simulink model "corripd"  (R2025b)
settings: Solver=ode5  StartTime=0.0  StopTime=2.335  FixedStep=0.001  MaxStep=0.001  RelTol=1e-3  AbsTol=1e-3
values from neighbouring files (symbols this model uses):
  b = 5E-5    (= 5e-05)    [Constants.m]
  J = 1    [Constants.m]
  Ka = 20    [Constants.m]
  Ki = 10000    [Constants.m]
  Km = 1.36    [Constants.m]
  Kp = 50    [Constants.m]
  Kv = Kvc    [Constants.m]
settings Model: ExtModeTrigMode=oneshot  ExtModeArmWhenConnect=off  Creator=Tomás  LastModifiedBy=Tomás
settings DataIOCC: SaveFormat=Array  SignalLoggingSaveFormat=ModelDataLogs  SaveOutput=off  SaveTime=off  ReturnWorkspaceOutputs=off
settings OptimizationCC: BlockReduction=off  BooleanDataType=off
settings DebuggingCC: SaveWithParameterizedLinksMsg=none  UnderspecifiedInitializationDetection=Classic  MergeDetectMultiDrivingBlocksExec=none  SignalResolutionControl=TryResolveAllWithWarning  MultiTaskDSMMsg=warning  MultiTaskCondExecSysMsg=none  UnconnectedInputMsg=warning  UnconnectedOutputMsg=warning  UnconnectedLineMsg=warning
settings HardwareCC: TargetUnknown=on
settings ModelReferenceCC: PropagateSignalLabelsOutOfModel=off
settings GRTTargetCC: CombineOutputUpdateFcns=off  GRTInterface=on

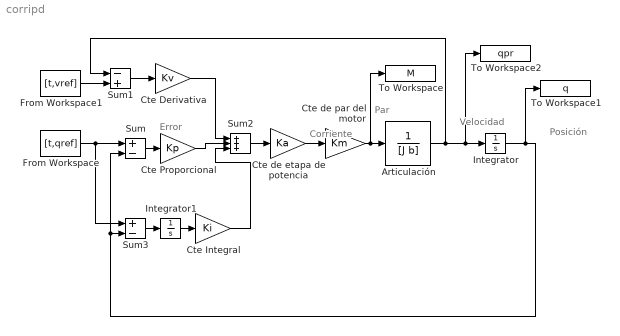
== system corripd ==
  note: Corriente
  note: Error
  note: Par
  note: Velocidad
  note: Posición
  Articulación : TransferFcn  Denominator=[J b]
  Cte Derivativa : Gain  Gain=Kv  SaturateOnIntegerOverflow=on  OutDataTypeStr=Inherit: Same as input  ParamDataTypeStr=Inherit: Same as input
  Cte Integral : Gain  Gain=Ki  SaturateOnIntegerOverflow=on  OutDataTypeStr=Inherit: Same as input  ParamDataTypeStr=Inherit: Same as input
  Cte Proporcional : Gain  Gain=Kp  SaturateOnIntegerOverflow=on  OutDataTypeStr=Inherit: Same as input  ParamDataTypeStr=Inherit: Same as input
  Cte de etapa de potencia : Gain  Gain=Ka  SaturateOnIntegerOverflow=on  OutDataTypeStr=Inherit: Same as input  ParamDataTypeStr=Inherit: Same as input
  Cte de par del motor : Gain  Gain=Km  SaturateOnIntegerOverflow=on  OutDataTypeStr=Inherit: Same as input  ParamDataTypeStr=Inherit: Same as input
  From Workspace : FromWorkspace  VariableName=[t,qref]  SampleTime=0.001  ZeroCross=off
  From Workspace1 : FromWorkspace  VariableName=[t,vref]  SampleTime=0.001  ZeroCross=off
  Integrator : Integrator
  Integrator1 : Integrator
  Sum : Sum  Inputs=+-  InputSameDT=on  SaturateOnIntegerOverflow=on  OutDataTypeStr=Inherit: Same as first input
  Sum1 : Sum  Inputs=-+  InputSameDT=on  SaturateOnIntegerOverflow=on  OutDataTypeStr=Inherit: Same as first input
  Sum2 : Sum  Inputs=+++  InputSameDT=on  SaturateOnIntegerOverflow=on  OutDataTypeStr=Inherit: Same as first input
  Sum3 : Sum  Inputs=+-  InputSameDT=on  SaturateOnIntegerOverflow=on  OutDataTypeStr=Inherit: Same as first input
  To Workspace : ToWorkspace  VariableName=M
      settings: MaxDataPoints=2335
  To Workspace1 : ToWorkspace  VariableName=q
      settings: MaxDataPoints=2335
  To Workspace2 : ToWorkspace  VariableName=qpr
      settings: MaxDataPoints=2335
  wires:
  Cte de etapa de potencia/1 -> Cte de par del motor/1
  From Workspace/1 -> Sum3/1, Sum/1
  Sum/1 -> Cte Proporcional/1
  Cte de par del motor/1 -> Articulación/1, To Workspace/1
  Sum1/1 -> Cte Derivativa/1
  From Workspace1/1 -> Sum1/2
  Cte Proporcional/1 -> Sum2/2
  Sum2/1 -> Cte de etapa de potencia/1
  Articulación/1 -> Integrator/1, To Workspace2/1, Sum1/1
  Cte Derivativa/1 -> Sum2/1
  Cte Integral/1 -> Sum2/3
  Integrator/1 -> Sum3/2, Sum/2, To Workspace1/1
  Sum3/1 -> Integrator1/1
  Integrator1/1 -> Cte Integral/1
